simulink model "jib_mpc"  (Simulink 7.9)
settings: Solver=VariableStepDiscrete  StartTime=0.0  StopTime=10.0  RelTol=1e-3
undefined symbols (not defined in the file or in its folder): jib, jib_x0, jib_xref, Ts
libraries: mpclib x1
settings Model: Creator=matias  LastModifiedBy=matias

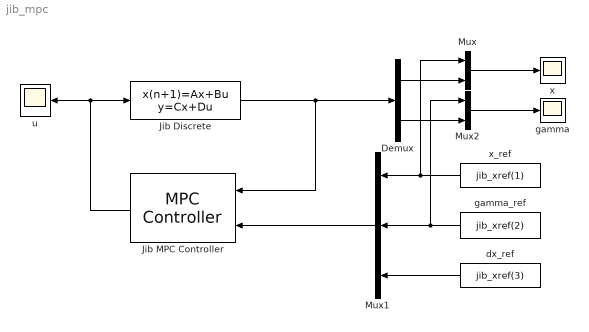
== system jib_mpc ==
  Demux : Demux  Outputs=2
  Jib Discrete : DiscreteStateSpace  A=jib.A  B=jib.B  C=jib.C(jib.OutputGroup.MO,:)  D=jib.D(jib.OutputGroup.MO,:)  X0=jib_x0  SampleTime=Ts
  Jib MPC Controller : mpclib/MPC Controller  mpcobj=jib_MPC  x0=[]  md_inport=off  mv_inport=off  lims_inport=off  switch_inport=off  ywt_inport=off  duwt_inport=off  rhoeps_inport=off  cost_outport=off  return_sequence=off  return_qpstatus=off  is_multiple=0  enable_value=0  n_mv=1  n_mo=2  n_md=0  n_ts=0.01  is_designfromscratch=0  ref_from_ws=off  ref_signal_name=[]  ref_preview=on  md_from_ws=off  md_signal_name=[]  md_preview=on  from_project=off  project_file=MPCtask.mat
  Mux : Mux  Inputs=2
  Mux1 : Mux  Inputs=3
  Mux2 : Mux  Inputs=2
  dx_ref : Constant  Value=jib_xref(3)
  gamma : Scope
      settings: SaveName=ScopeData2
  gamma_ref : Constant  Value=jib_xref(2)
  u : Scope
      settings: YMin=-350  YMax=350
  x : Scope
      settings: YMin=-7.5  YMax=0.5
  x_ref : Constant  Value=jib_xref(1)
  wires:
  Jib Discrete/1 -> Demux/1, Jib MPC Controller/1
  Jib MPC Controller/1 -> Jib Discrete/1, u/1
  Mux/1 -> x/1
  x_ref/1 -> Mux/1, Mux1/1
  Mux1/1 -> Jib MPC Controller/2
  Mux2/1 -> gamma/1
  Demux/1 -> Mux/2
  gamma_ref/1 -> Mux1/2, Mux2/1
  dx_ref/1 -> Mux1/3
  Demux/2 -> Mux2/2
